simulink model "ThisOne-merged"  (R2026a)
settings: Solver=ode3  StopTime=2  FixedStep=1e-6  EnableMultiTasking=on
PreLoadFcn:
  | BLDCSpeedControlData;
values from neighbouring files (symbols this model uses):
  Jm = 4.97    [BLDCSpeedControlDataNewParam.m]
  p = 4    [BLDCSpeedControlDataNewParam.m]
undefined symbols (not defined in the file or in its folder): Ct_CqToRPM, Down, Up
libraries: nesl_utility x13, fl_lib x9, ee_lib x5, eeGeneralControl x2, eeBldcCurrentController x1, batt_lib x1, slpidlib x1, SignalEditorBlockLib x1
(part 2 of 2)

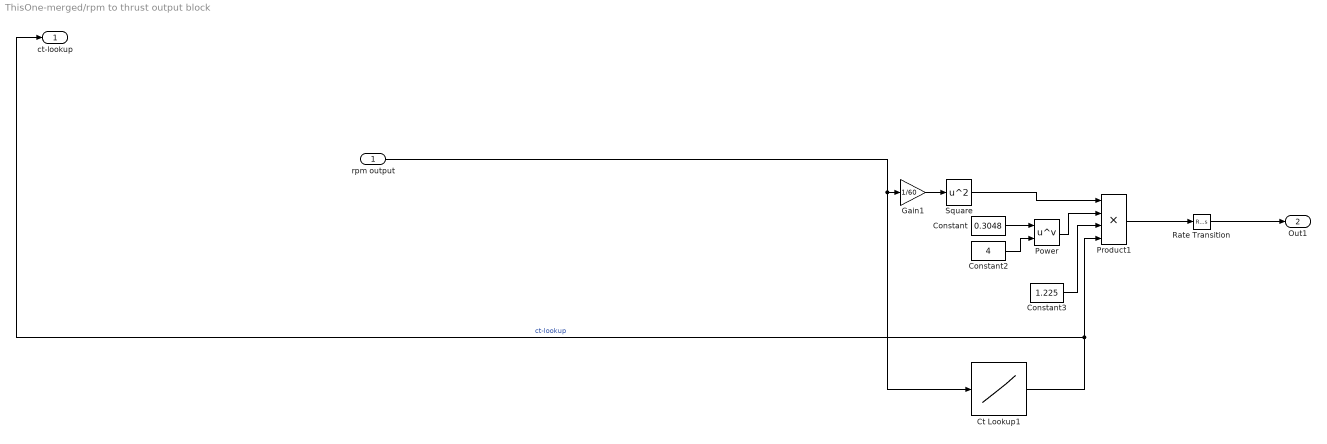
== system ThisOne-merged/rpm to thrust output block ==
  rpm output : Inport
  Constant : Constant  Value=0.3048
  Constant2 : Constant  Value=4
  Constant3 : Constant  Value=1.225
  Ct Lookup1 : Lookup_n-D  NumberOfTableDimensions=1  BreakpointsForDimension1=Ct_CqToRPM.RPM  Table=Ct_CqToRPM.Ct  InternalRulePriority=Speed  RndMeth=Simplest
  Gain1 : Gain  Gain=1/60
  Power : Math  Operator=pow
  Product1 : Product  Inputs=4
  Rate Transition : RateTransition
  Square : Math  Operator=square
  ct-lookup : Outport
  Out1 : Outport  Port=2
  wires:
  Constant3/1 -> Product1/3
  Square/1 -> Product1/1
  rpm output/1 -> Ct Lookup1/1, Gain1/1
  Constant2/1 -> Power/2
  Power/1 -> Product1/2
  Constant/1 -> Power/1
  Product1/1 -> Rate Transition/1
  Gain1/1 -> Square/1
  Ct Lookup1/1 -> ct-lookup/1, Product1/4  "ct-lookup"
  Rate Transition/1 -> Out1/1

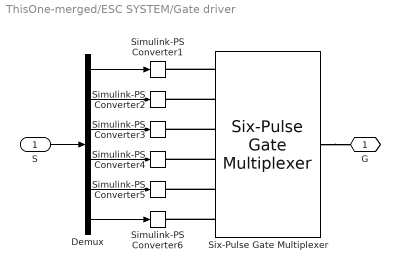
== system ThisOne-merged/ESC SYSTEM/Gate driver ==
  S : Inport
  Demux : Demux  Outputs=6
  Simulink-PS Converter{1..6} (6 alike) : nesl_utility/Simulink-PS Converter  PhysicalDomain=network_engine_domain  SubClassName=ps_input  LeftPortType=input  RightPortType=output  PseudoPeriodic=off  Frequencies=[]  NoiseDistribution=none  NoiseParameters=[]  Unit=1  AffineConversion=off  FilteringAndDerivatives=zero  SimscapeFilterOrder=1  InputFilterTimeConstant=0.001  UdotUserProvided=1
  Six-Pulse Gate Multiplexer : ee_lib/Semiconductors & Converters/Converters/Six-Pulse Gate Multiplexer  port_option=ee.enum.controlport.ps
  G : PMIOPort  Side=Right
  wires:
  Demux/1 -> Simulink-PS Converter1/1
  S/1 -> Demux/1
  Demux/4 -> Simulink-PS Converter4/1
  Demux/2 -> Simulink-PS Converter2/1
  Demux/3 -> Simulink-PS Converter3/1
  Demux/5 -> Simulink-PS Converter5/1
  Demux/6 -> Simulink-PS Converter6/1
  connections:
  Six-Pulse Gate Multiplexer/RConn1 -- G/RConn1
  Six-Pulse Gate Multiplexer/LConn6 -- Simulink-PS Converter6/RConn1
  Six-Pulse Gate Multiplexer/LConn5 -- Simulink-PS Converter5/RConn1
  Six-Pulse Gate Multiplexer/LConn4 -- Simulink-PS Converter4/RConn1
  Six-Pulse Gate Multiplexer/LConn3 -- Simulink-PS Converter3/RConn1
  Six-Pulse Gate Multiplexer/LConn2 -- Simulink-PS Converter2/RConn1
  Six-Pulse Gate Multiplexer/LConn1 -- Simulink-PS Converter1/RConn1

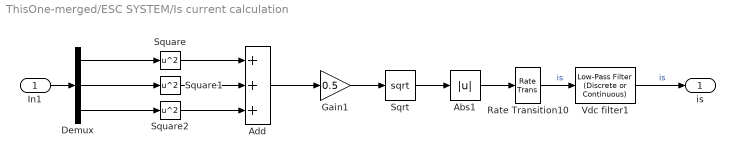
== system ThisOne-merged/ESC SYSTEM/Is current calculation ==
  In1 : Inport
  Abs1 : Abs  SaturateOnIntegerOverflow=off
  Add : Sum  Inputs=+++
  Demux : Demux  Outputs=3
  Gain1 : Gain  Gain=0.5
  Rate Transition10 : RateTransition
  Sqrt : Sqrt
  Square : Math  Operator=square
  Square1 : Math  Operator=square
  Square2 : Math  Operator=square
  Vdc filter1 : eeGeneralControl/Low-Pass Filter (Discrete or Continuous)  K=1  T=0.005  B=inf  A=-inf  init_option=Inherited from block input  x0=0  Ts=1e-5
  is : Outport
  wires:
  Rate Transition10/1 -> Vdc filter1/1  "is"
  Demux/1 -> Square/1
  Abs1/1 -> Rate Transition10/1
  Sqrt/1 -> Abs1/1
  Add/1 -> Gain1/1
  Vdc filter1/1 -> is/1  "is"
  Square1/1 -> Add/2
  Gain1/1 -> Sqrt/1
  Demux/2 -> Square1/1
  Demux/3 -> Square2/1
  Square/1 -> Add/1
  Square2/1 -> Add/3
  In1/1 -> Demux/1

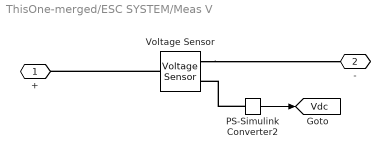
== system ThisOne-merged/ESC SYSTEM/Meas V ==
  PS-Simulink Converter2 : nesl_utility/PS-Simulink Converter  PhysicalDomain=network_engine_domain  SubClassName=ps_output  LeftPortType=input  RightPortType=output  PseudoPeriodic=off  Frequencies=[]  VectorFormat=1-D array  Unit=V  AffineConversion=off
  Voltage Sensor : fl_lib/Electrical/Electrical Sensors/Voltage Sensor
  + : PMIOPort  Side=Left
  - : PMIOPort  Port=2  Side=Right
  tag scope: Vdc=global
  wires:
  PS-Simulink Converter2/1 -> [Vdc]
  connections:
  Voltage Sensor/LConn1 -- +/RConn1
  PS-Simulink Converter2/LConn1 -- Voltage Sensor/RConn1
  Voltage Sensor/RConn2 -- -/RConn1

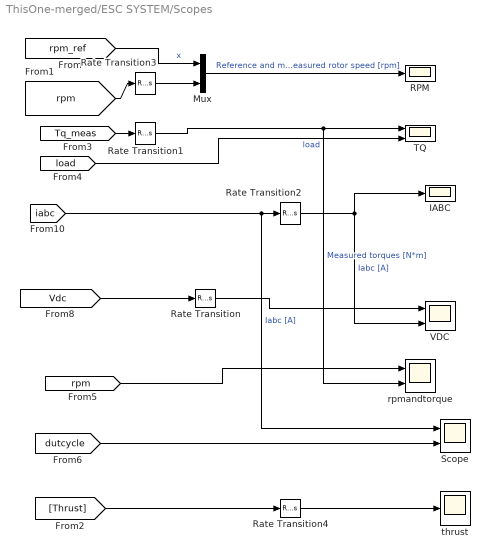
== system ThisOne-merged/ESC SYSTEM/Scopes ==
  IABC : Scope
      settings: ActiveDisplayYMinimum=-3.7631805549135566  ActiveDisplayYMaximum=3.2616947486453842  DataLoggingSaveFormat=Array
  Mux : Mux  Inputs=2
  RPM : Scope
      settings: ActiveDisplayYMinimum=4423.2627511819474  ActiveDisplayYMaximum=4982.0373549791029  DataLoggingVariableName=ScopeData5  DataLoggingSaveFormat=Array
  Rate Transition{,1,3..4} (4 alike) : RateTransition
  Rate Transition2 : RateTransition  OutPortSampleTime=1e-4
  Scope : Scope  NumInputPorts=2
      settings: ActiveDisplayYMinimum=-3.1325027281177791  ActiveDisplayYMaximum=3.1274558958611394
  TQ : Scope  NumInputPorts=2
      settings: ActiveDisplayYMinimum=-0.026277929525903816  ActiveDisplayYMaximum=0.0058519977724514165  DataLoggingVariableName=ScopeData7  DataLoggingSaveFormat=Array
  VDC : Scope  NumInputPorts=2
      settings: ActiveDisplayYMinimum=8.2547903144741781  ActiveDisplayYMaximum=59.260482079430432  DataLoggingVariableName=ScopeData8  DataLoggingSaveFormat=Array
  rpmandtorque : Scope  NumInputPorts=2
      settings: ActiveDisplayYMinimum=-0.026277929525903816  ActiveDisplayYMaximum=0.0058519977724514165  DataLoggingVariableName=ScopeData10
  thrust : Scope
      settings: ActiveDisplayYMinimum=-2.0635196043153279  ActiveDisplayYMaximum=8.8562754165520339  DataLoggingVariableName=ScopeData9
  wires:
  [rpm] -> Rate Transition3/1
  [iabc] -> Scope/1, Rate Transition2/1  "Iabc [A]"
  [rpm_ref] -> Mux/1  "x"
  [Tq_meas] -> Rate Transition1/1
  Rate Transition1/1 -> rpmandtorque/2, TQ/1  "Measured torques [N*m]"
  Mux/1 -> RPM/1  "Reference and measured rotor speed [rpm]"
  [load] -> TQ/2  "load"
  Rate Transition3/1 -> Mux/2
  [rpm] -> rpmandtorque/1
  [Vdc] -> Rate Transition/1
  Rate Transition/1 -> VDC/1
  Rate Transition2/1 -> VDC/2, IABC/1  "Iabc [A]"
  [dutcycle] -> Scope/2
  [Thrust] -> Rate Transition4/1
  Rate Transition4/1 -> thrust/1

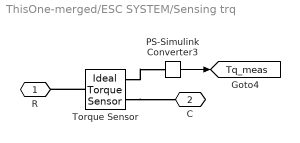
== system ThisOne-merged/ESC SYSTEM/Sensing trq ==
  PS-Simulink Converter3 : nesl_utility/PS-Simulink Converter  PhysicalDomain=network_engine_domain  SubClassName=ps_output  LeftPortType=input  RightPortType=output  PseudoPeriodic=off  Frequencies=[]  VectorFormat=1-D array  Unit=N*m  AffineConversion=off
  Torque Sensor : fl_lib/Mechanical/Mechanical Sensors/Ideal Torque Sensor
  R : PMIOPort  Side=Left
  C : PMIOPort  Port=2  Side=Right
  tag scope: Tq_meas=global
  wires:
  PS-Simulink Converter3/1 -> [Tq_meas]
  connections:
  Torque Sensor/RConn1 -- C/RConn1
  Torque Sensor/RConn2 -- PS-Simulink Converter3/LConn1
  Torque Sensor/LConn1 -- R/RConn1

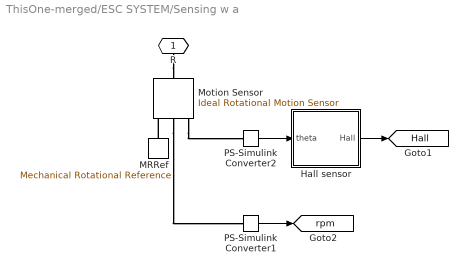
== system ThisOne-merged/ESC SYSTEM/Sensing w a ==
  Hall sensor : Subsystem
  MRRef : fl_lib/Mechanical/Rotational Elements/Mechanical Rotational Reference
  Motion Sensor : fl_lib/Mechanical/Mechanical Sensors/Ideal Rotational Motion Sensor  reference=foundation.enum.MeasurementReference.difference  acceleration_port=false  velocity_port=true  position_port=true  wrap_angle=false  offset=0 deg
  PS-Simulink Converter1 : nesl_utility/PS-Simulink Converter  PhysicalDomain=network_engine_domain  SubClassName=ps_output  LeftPortType=input  RightPortType=output  PseudoPeriodic=off  Frequencies=[]  VectorFormat=1-D array  Unit=rpm  AffineConversion=off
  PS-Simulink Converter2 : nesl_utility/PS-Simulink Converter  PhysicalDomain=network_engine_domain  SubClassName=ps_output  LeftPortType=input  RightPortType=output  PseudoPeriodic=off  Frequencies=[]  VectorFormat=1-D array  Unit=rad  AffineConversion=off
  R : PMIOPort  Side=Left
  tag scope: Hall=global, rpm=global
  wires:
  PS-Simulink Converter1/1 -> [rpm]
  PS-Simulink Converter2/1 -> Hall sensor/1(theta)
  Hall sensor/1(Hall) -> [Hall]
  connections:
  R/RConn1 -- Motion Sensor/LConn1
  Motion Sensor/RConn2 -- PS-Simulink Converter1/LConn1
  MRRef/LConn1 -- Motion Sensor/RConn1
  Motion Sensor/RConn3 -- PS-Simulink Converter2/LConn1

== system ThisOne-merged/ESC SYSTEM/Sensing iabc ==
  Current Sensor : ee_lib/Sensors & Transducers/Current Sensor (Three-Phase)  port_option=ee.enum.threePhasePort.composite
  PS-Simulink Converter : nesl_utility/PS-Simulink Converter  PhysicalDomain=network_engine_domain  SubClassName=ps_output  LeftPortType=input  RightPortType=output  PseudoPeriodic=off  Frequencies=[]  VectorFormat=1-D array  Unit=A  AffineConversion=off
  1 : PMIOPort  Side=Left
  2 : PMIOPort  Port=2  Side=Right
  tag scope: iabc=global
  wires:
  PS-Simulink Converter/1 -> [iabc]
  connections:
  1/RConn1 -- Current Sensor/LConn1
  2/RConn1 -- Current Sensor/RConn2
  Current Sensor/RConn1 -- PS-Simulink Converter/LConn1

== system ThisOne-merged/ESC SYSTEM/Sign ==
  u : Inport
  Constant2 : Constant
  Constant3 : Constant  Value=-1
  Switch : Switch  SaturateOnIntegerOverflow=off  InputSameDT=off
  y : Outport
  wires:
  Constant3/1 -> Switch/3
  Constant2/1 -> Switch/1
  u/1 -> Switch/2
  Switch/1 -> y/1

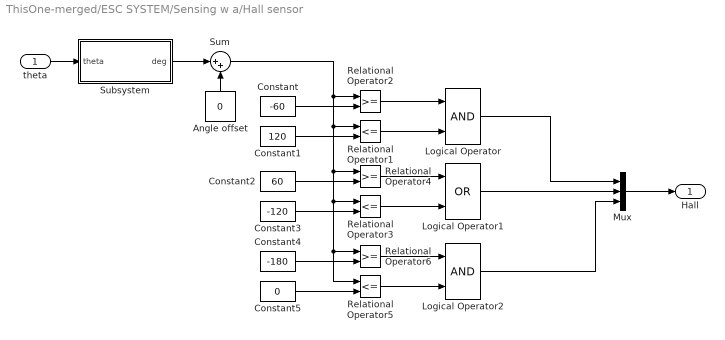
== system ThisOne-merged/ESC SYSTEM/Sensing w a/Hall sensor ==
  theta : Inport
  Angle offset : Constant  Value=0
  Constant : Constant  Value=-60
  Constant1 : Constant  Value=120
  Constant2 : Constant  Value=60
  Constant3 : Constant  Value=-120
  Constant4 : Constant  Value=-180
  Constant5 : Constant  Value=0
  Logical Operator : Logic  AllPortsSameDT=off  OutDataTypeStr=boolean
  Logical Operator1 : Logic  Operator=OR  AllPortsSameDT=off  OutDataTypeStr=boolean
  Logical Operator2 : Logic  AllPortsSameDT=off  OutDataTypeStr=boolean
  Mux : Mux  Inputs=3
  Relational Operator1 : RelationalOperator  Operator=<=
  Relational Operator2 : RelationalOperator
  Relational Operator3 : RelationalOperator  Operator=<=
  Relational Operator4 : RelationalOperator
  Relational Operator5 : RelationalOperator  Operator=<=
  Relational Operator6 : RelationalOperator
  Subsystem : Subsystem
  Sum : Sum  Inputs=|++
  Hall : Outport  VectorParamsAs1DForOutWhenUnconnected=off
  wires:
  Constant3/1 -> Relational Operator3/2
  Logical Operator2/1 -> Mux/3
  Logical Operator1/1 -> Mux/2
  Logical Operator/1 -> Mux/1
  Relational Operator5/1 -> Logical Operator2/2
  Relational Operator6/1 -> Logical Operator2/1
  Constant4/1 -> Relational Operator6/2
  Constant5/1 -> Relational Operator5/2
  Relational Operator3/1 -> Logical Operator1/2
  Mux/1 -> Hall/1
  Relational Operator2/1 -> Logical Operator/1
  Relational Operator1/1 -> Logical Operator/2
  Constant/1 -> Relational Operator2/2
  Relational Operator4/1 -> Logical Operator1/1
  Constant1/1 -> Relational Operator1/2
  Constant2/1 -> Relational Operator4/2
  theta/1 -> Subsystem/1(theta)
  Subsystem/1(deg) -> Sum/1
  Sum/1 -> Relational Operator1/1, Relational Operator5/1, Relational Operator6/1, Relational Operator3/1, Relational Operator4/1, Relational Operator2/1
  Angle offset/1 -> Sum/2

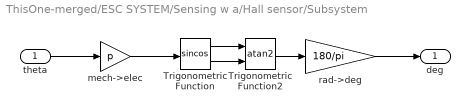
== system ThisOne-merged/ESC SYSTEM/Sensing w a/Hall sensor/Subsystem ==
  theta : Inport
  Trigonometric Function : Trigonometry  Operator=sincos
  Trigonometric Function2 : Trigonometry  Operator=atan2
  mech->elec : Gain  Gain=p
  rad->deg : Gain  Gain=180/pi  SaturateOnIntegerOverflow=on  OutDataTypeStr=Inherit: Same as input  ParamDataTypeStr=Inherit: Same as input
  deg : Outport  VectorParamsAs1DForOutWhenUnconnected=off
  wires:
  Trigonometric Function2/1 -> rad->deg/1
  Trigonometric Function/1 -> Trigonometric Function2/1
  theta/1 -> mech->elec/1
  rad->deg/1 -> deg/1
  Trigonometric Function/2 -> Trigonometric Function2/2
  mech->elec/1 -> Trigonometric Function/1
